simulink model "Inverter"  (Simulink 8.3)
settings: Solver=ode45  StartTime=0.0  StopTime=tfin  RelTol=1e-3
values from neighbouring files (symbols this model uses):
  Bridge_Inductances = 4e-3    (= 0.004)    [Inverter_ini.m]
  Buffer_Capacitance = 10e-3    (= 0.01)    [Inverter_ini.m]
  sample = 10e-5    (= 0.0001)    [Inverter_ini.m]    (also in Sketch_controller_model_ini.m; Symmetry_REAL_TIME_ini.m; Symmetry_ini.m; Symmetry_ini_COPY.m)
undefined symbols (not defined in the file or in its folder): Ion, Lithium
libraries: powerlib x69, simulink x5, dspsigops x4, dsparch4 x2, electricdrivelib x1
settings Model: Creator=gorbep  LastModifiedBy=Templomos
settings DataIOCC: SignalLoggingSaveFormat=Dataset
settings DebuggingCC: UnderspecifiedInitializationDetection=Simplified  StateNameClashWarn=none
settings GRTTargetCC: CombineOutputUpdateFcns=on  GRTInterface=off

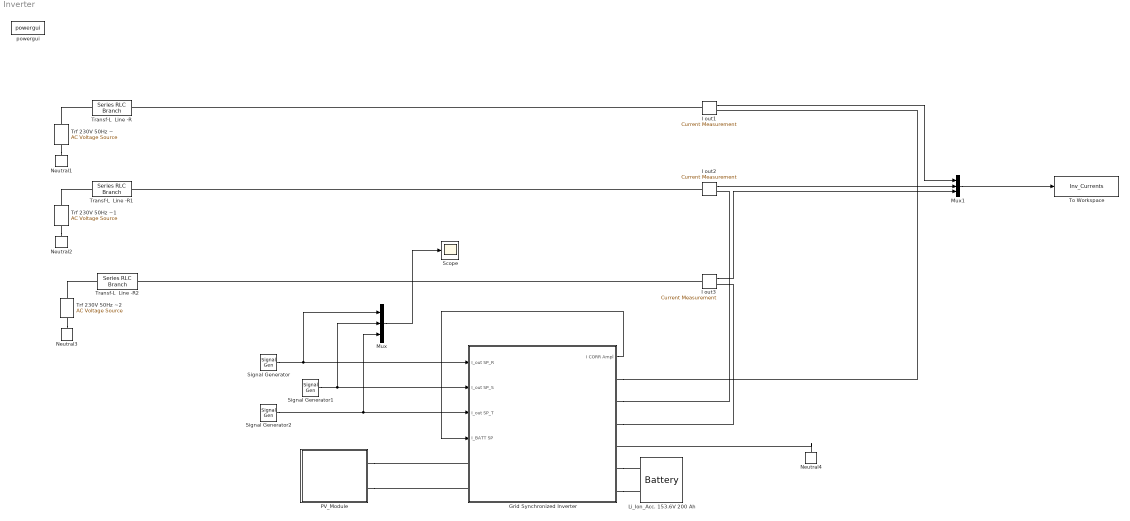
== system Inverter ==
  Grid Synchronized Inverter : Subsystem
  I out1 : powerlib/Measurements/Current Measurement  PhasorSimulation=off  OutputType=Complex  PSBequivalent=0
  I out2 : powerlib/Measurements/Current Measurement  PhasorSimulation=off  OutputType=Complex  PSBequivalent=0
  I out3 : powerlib/Measurements/Current Measurement  PhasorSimulation=off  OutputType=Complex  PSBequivalent=0
  Li_Ion_Acc. 153.6V 200 Ah : electricdrivelib/Extra Sources/Battery  BatType=Lithium-Ion  ShowDetailedParameters=off  NomV=153.6  NomQ=200  SOC=50  PresetModel=off  MaxQ=210  FullV=274.6189824  Dis_rate=173.913  R=0.00768  Normal_OP=361.7392  expZone=[254.8950528 19.652174]  Dis_Char=off  current=[1.5 3]  Units=Ampere-hour  Batt_Tr=30
  Mux : Mux  Inputs=3
  Mux1 : Mux  Inputs=3
  Neutral{1..4} (4 alike) : powerlib/Elements/Neutral  LConnTagsString=a  NodeNumber=10
  PV_Module : Subsystem
  Scope : Scope
      settings: SaveName=ScopeData5
  Signal Generator : SignalGenerator  WaveForm=sawtooth  Frequency=200
  Signal Generator1 : SignalGenerator  WaveForm=square  Frequency=200
  Signal Generator2 : SignalGenerator  Frequency=200
  To Workspace : ToWorkspace  VariableName=Inv_Currents  SaveFormat=Structure With Time  SampleTime=sample
  Transf-L  Line -R : powerlib/Elements/Series RLC Branch  LConnTagsString=__new0  RConnTagsString=__new0  BranchType=RL  Resistance=0.01  Inductance=0  SetiL0=off  InitialCurrent=0  Capacitance=1.0  Setx0=off  InitialVoltage=0  Measurements=None
  Transf-L  Line -R1 : powerlib/Elements/Series RLC Branch  LConnTagsString=__new0  RConnTagsString=__new0  BranchType=RL  Resistance=0.01  Inductance=0  SetiL0=off  InitialCurrent=0  Capacitance=1.0  Setx0=off  InitialVoltage=0  Measurements=None
  Transf-L  Line -R2 : powerlib/Elements/Series RLC Branch  LConnTagsString=__new0  RConnTagsString=__new0  BranchType=RL  Resistance=0.01  Inductance=0  SetiL0=off  InitialCurrent=0  Capacitance=1.0  Setx0=off  InitialVoltage=0  Measurements=None
  Trf 230V 50Hz ~ : powerlib/Electrical Sources/AC Voltage Source  Amplitude=325.2691  Phase=0  Frequency=50  SampleTime=0  Measurements=None
  Trf 230V 50Hz ~1 : powerlib/Electrical Sources/AC Voltage Source  Amplitude=325.2691  Phase=-120  Frequency=50  SampleTime=0  Measurements=None
  Trf 230V 50Hz ~2 : powerlib/Electrical Sources/AC Voltage Source  Amplitude=325.2691  Phase=-240  Frequency=50  SampleTime=0  Measurements=None
  powergui : powerlib/powergui  SimulationMode=Continuous  SolverType=Tustin  SampleTime=50e-6  frequency=60  SPID=off  DisableSnubberDevices=off  DisableRonSwitches=off  DisableVfSwitches=off  SwTol=0  Interpol=off  DisplayEquations=off  Ts=0  methode=off  frequencyindice=50  Pbase=100e6  ErrMax=1e-4  Iterations=50  UnitsV=kV  UnitsW=MW  FunctionMessages=off  echomessages=off  HookPort=off  EnableUseOfTLC=off  x0status=blocks  RestoreLinks=warning  ResistiveCurrentMeasurement=off  Frange=[0:2:500]  Ylog=off  Xlog=on  ShowGrid=off  save=off  variable=ZData  structure=0  ZoomFFT=on  StartTime=0.0  cycles=1  DisplayStyle=1  fundamental=60  FreqAxis=off  MaxFrequency=1000  frequencyindicesteady=1  RmsSteady=1  display=off
  wires:
  Grid Synchronized Inverter/1(I CORR Ampl) -> Grid Synchronized Inverter/4(I_BATT SP)
  Signal Generator/1 -> Mux/1, Grid Synchronized Inverter/1(I_out SP_R)
  Signal Generator1/1 -> Mux/2, Grid Synchronized Inverter/2(I_out SP_S)
  Signal Generator2/1 -> Mux/3, Grid Synchronized Inverter/3(I_out SP_T)
  I out1/1 -> Mux1/1
  I out2/1 -> Mux1/2
  I out3/1 -> Mux1/3
  Mux1/1 -> To Workspace/1
  Mux/1 -> Scope/1
  connections:
  Grid Synchronized Inverter/RConn5 -- Li_Ion_Acc. 153.6V 200 Ah/LConn1
  Grid Synchronized Inverter/RConn6 -- Li_Ion_Acc. 153.6V 200 Ah/LConn2
  Transf-L  Line -R/LConn1 -- Trf 230V 50Hz ~/RConn1
  Trf 230V 50Hz ~/LConn1 -- Neutral1/LConn1
  Transf-L  Line -R1/LConn1 -- Trf 230V 50Hz ~1/RConn1
  Trf 230V 50Hz ~1/LConn1 -- Neutral2/LConn1
  Trf 230V 50Hz ~2/LConn1 -- Neutral3/LConn1
  Transf-L  Line -R2/LConn1 -- Trf 230V 50Hz ~2/RConn1
  I out1/LConn1 -- Transf-L  Line -R/RConn1
  I out2/LConn1 -- Transf-L  Line -R1/RConn1
  I out3/LConn1 -- Transf-L  Line -R2/RConn1
  Neutral4/LConn1 -- Grid Synchronized Inverter/RConn4
  Grid Synchronized Inverter/RConn1 -- I out1/RConn1
  Grid Synchronized Inverter/RConn2 -- I out2/RConn1
  Grid Synchronized Inverter/RConn3 -- I out3/RConn1
  PV_Module/RConn1 -- Grid Synchronized Inverter/LConn1
  PV_Module/RConn2 -- Grid Synchronized Inverter/LConn2

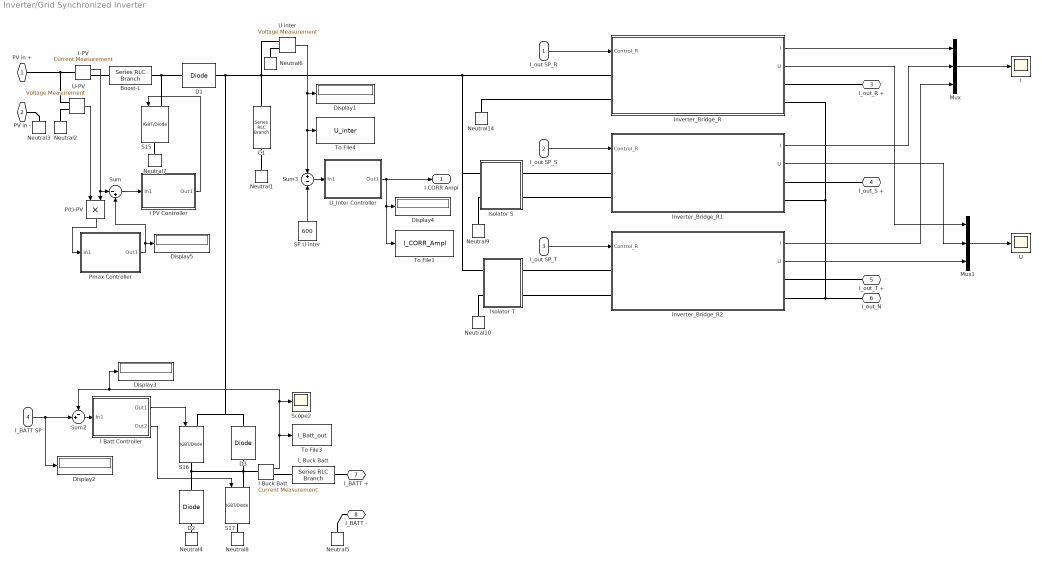
== system Inverter/Grid Synchronized Inverter ==
  I_out SP_R : Inport
  I_out SP_S : Inport  Port=2
  I_out SP_T : Inport  Port=3
  I_BATT SP : Inport  Port=4
  " Boost-L" : powerlib/Elements/Series RLC Branch  LConnTagsString=__new0  RConnTagsString=__new0  BranchType=L  Resistance=8  Inductance=100e-3  SetiL0=off  InitialCurrent=30  Capacitance=1.0  Setx0=off  InitialVoltage=0  Measurements=None
  C1 : powerlib/Elements/Series RLC Branch  LConnTagsString=__new0  RConnTagsString=__new0  BranchType=C  Resistance=35.35  Inductance=0.1125  SetiL0=off  InitialCurrent=0  Capacitance=Buffer_Capacitance  Setx0=on  InitialVoltage=Buffer_Initial_Voltage  Measurements=None
  D1 : powerlib/Power Electronics/Diode  Ron=0.001  Lon=0  Vf=0.8  IC=0  UseSnubber=off  Rs=50000  Cs=250e-9  Measurements=off
  D2 : powerlib/Power Electronics/Diode  Ron=0.001  Lon=0  Vf=0.8  IC=0  UseSnubber=off  Rs=50000  Cs=250e-9  Measurements=off
  D3 : powerlib/Power Electronics/Diode  Ron=0.001  Lon=0  Vf=0.8  IC=0  UseSnubber=off  Rs=50000  Cs=250e-9  Measurements=off
  Display{1..5} (5 alike) : Display
  I : Scope
      settings: YMin=-550  YMax=400
  I Batt Controller : Subsystem
  I Buck Batt : powerlib/Measurements/Current Measurement  PhasorSimulation=off  OutputType=Complex  PSBequivalent=0
  I PV Controller : Subsystem
  I-PV : powerlib/Measurements/Current Measurement  PhasorSimulation=off  OutputType=Complex  PSBequivalent=0
  Inverter_Bridge_R : Subsystem
  Inverter_Bridge_R1 : Subsystem
  Inverter_Bridge_R2 : Subsystem
  Isolator S : Subsystem
  Isolator T : Subsystem
  L Buck Batt : powerlib/Elements/Series RLC Branch  LConnTagsString=__new0  RConnTagsString=__new0  BranchType=L  Resistance=100  Inductance=1e-1  SetiL0=on  InitialCurrent=0  Capacitance=1.0  Setx0=off  InitialVoltage=0  Measurements=None
  Mux : Mux  Inputs=3
  Mux1 : Mux  Inputs=3
  Neutral{1..10,14} (11 alike) : powerlib/Elements/Neutral  LConnTagsString=a  NodeNumber=1
  P(t)-PV : Product  RndMeth=Zero
  Pmax Controller : Subsystem
  S15 : powerlib/Power Electronics/IGBT//Diode  Ron=1e-3  Rs=1e5  Cs=inf  Measurements=off
  S16 : powerlib/Power Electronics/IGBT//Diode  Ron=1e-3  Rs=1e5  Cs=inf  Measurements=off
  S17 : powerlib/Power Electronics/IGBT//Diode  Ron=1e-3  Rs=1e5  Cs=inf  Measurements=off
  SP U inter : Constant  Value=600
  Scope2 : Scope
      settings: TimeRange=0.1  YMin=-40  YMax=40  SaveName=ScopeData2
  Sum : Sum  Inputs=|-+
  Sum2 : Sum  Inputs=-+|
  Sum3 : Sum  Inputs=+-
  To File1 : ToFile  Filename=I_CORR_Ampl  MatrixName=y  SampleTime=5e-3
  To File3 : ToFile  Filename=I_Batt_out  MatrixName=y  SampleTime=5e-3
  To File4 : ToFile  Filename=U_inter  MatrixName=y  SampleTime=5e-3
  U : Scope
      settings: YMin=-1.1  YMax=1.1
  U inter : powerlib/Measurements/Voltage Measurement  PhasorSimulation=off  OutputType=Complex  PSBequivalent=0
  U-PV : powerlib/Measurements/Voltage Measurement  PhasorSimulation=off  OutputType=Complex  PSBequivalent=0
  U_Inter Controller : Subsystem
  " PV in +" : PMIOPort  Port=1  Side=Left
  " PV in -" : PMIOPort  Port=2  Side=Left
  " I_out_R +" : PMIOPort  Port=3  Side=Right
  " I_out_S +" : PMIOPort  Port=4  Side=Right
  " I_out_T +" : PMIOPort  Port=5  Side=Right
  " I_out_N" : PMIOPort  Port=6  Side=Right
  " I_BATT +" : PMIOPort  Port=7  Side=Right
  " I_BATT -" : PMIOPort  Port=8  Side=Right
  I CORR Ampl : Outport
  wires:
  U inter/1 -> Sum3/1, To File4/1, Display1/1
  Sum/1 -> I PV Controller/1(In1)
  I-PV/1 -> Sum/1, P(t)-PV/2
  SP U inter/1 -> Sum3/2
  U-PV/1 -> P(t)-PV/1
  Pmax Controller/1(Out1) -> Display5/1, Sum/2
  I PV Controller/1(Out1) -> S15/1
  P(t)-PV/1 -> Pmax Controller/1(In1)
  U_Inter Controller/1(Out1) -> I CORR Ampl/1, To File1/1, Display4/1
  Sum3/1 -> U_Inter Controller/1(In1)
  Sum2/1 -> I Batt Controller/1(In1)
  I Buck Batt/1 -> To File3/1, Scope2/1, Sum2/1, Display3/1
  I Batt Controller/1(Out1) -> S16/1
  I_BATT SP/1 -> Sum2/2, Display2/1
  I Batt Controller/2(Out2) -> S17/1
  I_out SP_R/1 -> Inverter_Bridge_R/1(Control_R)
  I_out SP_S/1 -> Inverter_Bridge_R1/1(Control_R)
  I_out SP_T/1 -> Inverter_Bridge_R2/1(Control_R)
  Inverter_Bridge_R/1(I) -> Mux/1
  Inverter_Bridge_R1/1(I) -> Mux/2
  Inverter_Bridge_R2/1(I) -> Mux/3
  Mux1/1 -> U/1
  Inverter_Bridge_R2/2(U) -> Mux1/3
  Inverter_Bridge_R1/2(U) -> Mux1/2
  Inverter_Bridge_R/2(U) -> Mux1/1
  Mux/1 -> I/1
  connections:
  " Boost-L"/RConn1 -- D1/LConn1 -- S15/LConn1
  " PV in +"/RConn1 -- I-PV/LConn1 -- U-PV/LConn1
  Neutral6/LConn1 -- U inter/LConn2
  Neutral7/LConn1 -- S15/RConn1
  I-PV/RConn1 -- " Boost-L"/LConn1
  Neutral1/LConn1 -- C1/RConn1
  U-PV/LConn2 -- Neutral2/LConn1
  " PV in -"/RConn1 -- Neutral3/LConn1
  I Buck Batt/LConn1 -- S17/LConn1 -- D3/LConn1 -- S16/RConn1 -- D2/RConn1
  Neutral4/LConn1 -- D2/LConn1
  L Buck Batt/RConn1 -- " I_BATT +"/RConn1
  Neutral5/LConn1 -- " I_BATT -"/RConn1
  S17/RConn1 -- Neutral8/LConn1
  I Buck Batt/RConn1 -- L Buck Batt/LConn1
  C1/LConn1 -- Isolator T/RConn1 -- Isolator S/RConn1 -- Inverter_Bridge_R/LConn1 -- D3/RConn1 -- S16/LConn1 -- D1/RConn1 -- U inter/LConn1
  Neutral10/LConn1 -- Isolator T/RConn2
  Neutral9/LConn1 -- Isolator S/RConn2
  " I_out_R +"/RConn1 -- Inverter_Bridge_R/RConn1
  Inverter_Bridge_R/LConn2 -- Neutral14/LConn1
  Inverter_Bridge_R1/LConn1 -- Isolator S/LConn1
  Inverter_Bridge_R1/LConn2 -- Isolator S/LConn2
  Inverter_Bridge_R1/RConn1 -- " I_out_S +"/RConn1
  " I_out_N"/RConn1 -- Inverter_Bridge_R2/RConn2 -- Inverter_Bridge_R1/RConn2 -- Inverter_Bridge_R/RConn2
  Inverter_Bridge_R2/LConn1 -- Isolator T/LConn1
  Inverter_Bridge_R2/LConn2 -- Isolator T/LConn2
  Inverter_Bridge_R2/RConn1 -- " I_out_T +"/RConn1

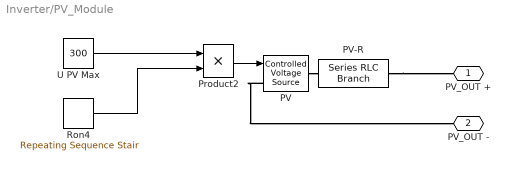
== system Inverter/PV_Module ==
  PV : powerlib/Electrical Sources/Controlled Voltage Source  Initialize=off  Source_Type=AC  Amplitude=0  Phase=0  Frequency=0  Measurements=None
  PV-R : powerlib/Elements/Series RLC Branch  LConnTagsString=__new0  RConnTagsString=__new0  BranchType=R  Resistance=5  Inductance=0.1  SetiL0=off  InitialCurrent=0  Capacitance=1.0  Setx0=off  InitialVoltage=0  Measurements=None
  Product2 : Product  RndMeth=Zero
  Ron4 : simulink/Sources/Repeating Sequence Stair  OutValues=[1 1 0 0].'  tsamp=0.5  OutMin=[]  OutMax=[]  OutDataTypeStr=float('double')  OutputDataTypeScalingMode=Specify via dialog  OutDataType=float('double')  ConRadixGroup=Best Precision: Vector-wise  OutScaling=2^-12
  U PV Max : Constant  Value=300
  PV_OUT + : PMIOPort  Port=1  Side=Right
  PV_OUT - : PMIOPort  Port=2  Side=Right
  wires:
  Product2/1 -> PV/1
  U PV Max/1 -> Product2/1
  Ron4/1 -> Product2/2
  connections:
  PV/LConn1 -- PV_OUT -/RConn1
  PV/RConn1 -- PV-R/LConn1
  PV-R/RConn1 -- PV_OUT +/RConn1

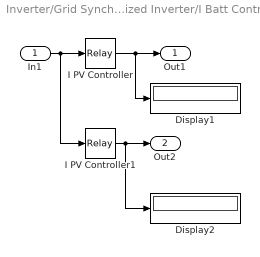
== system Inverter/Grid Synchronized Inverter/I Batt Controller ==
  In1 : Inport
  Display1 : Display
  Display2 : Display
  I PV Controller : Relay  OnSwitchValue=0.01  OffSwitchValue=-0.01  ZeroCross=off  SampleTime=1e-4
  I PV Controller1 : Relay  OnSwitchValue=0.01  OffSwitchValue=-0.01  OnOutputValue=0  OffOutputValue=1  ZeroCross=off  SampleTime=1e-4
  Out1 : Outport
  Out2 : Outport  Port=2
  wires:
  In1/1 -> I PV Controller/1, I PV Controller1/1
  I PV Controller/1 -> Out1/1, Display1/1
  I PV Controller1/1 -> Out2/1, Display2/1

== system Inverter/Grid Synchronized Inverter/I PV Controller ==
  In1 : Inport
  I PV Controller : Relay  OnSwitchValue=0.01  OffSwitchValue=-0.01  ZeroCross=off  SampleTime=1e-4
  Out1 : Outport
  wires:
  In1/1 -> I PV Controller/1
  I PV Controller/1 -> Out1/1

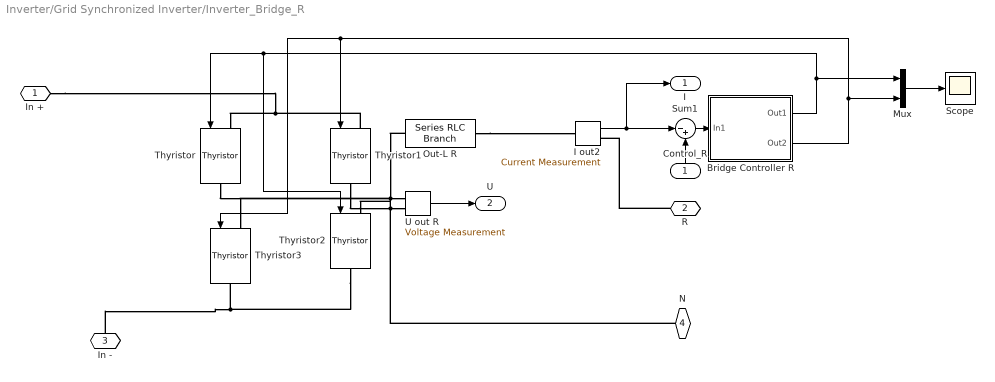
== system Inverter/Grid Synchronized Inverter/Inverter_Bridge_R ==
  Control_R : Inport
  " Out-L R" : powerlib/Elements/Series RLC Branch  LConnTagsString=__new0  RConnTagsString=__new0  BranchType=L  Resistance=100  Inductance=Bridge_Inductances  SetiL0=off  InitialCurrent=0  Capacitance=1.0  Setx0=off  InitialVoltage=0  Measurements=None
  Bridge Controller R : Subsystem
  I out2 : powerlib/Measurements/Current Measurement  PhasorSimulation=off  OutputType=Complex  PSBequivalent=0
  Mux : Mux  Inputs=2
  Scope : Scope
      settings: SaveName=ScopeData4
  Sum1 : Sum  Inputs=|-+
  Thyristor{,1..3} (4 alike) : powerlib/Power Electronics/Thyristor  Ron=1e-3  Lon=0  Vf=0.8  IC=0  Rs=500  Cs=inf  Measurements=off
  U out R : powerlib/Measurements/Voltage Measurement  PhasorSimulation=off  OutputType=Complex  PSBequivalent=0
  In + : PMIOPort  Port=1  Side=Left
  R : PMIOPort  Port=2  Side=Right
  In - : PMIOPort  Port=3  Side=Left
  N : PMIOPort  Port=4  Side=Right
  I : Outport
  U : Outport  Port=2
  wires:
  I out2/1 -> I/1, Sum1/1
  Bridge Controller R/2(Out2) -> Mux/2, Thyristor1/1, Thyristor3/1
  Bridge Controller R/1(Out1) -> Mux/1, Thyristor2/1, Thyristor/1
  Sum1/1 -> Bridge Controller R/1(In1)
  Control_R/1 -> Sum1/2
  U out R/1 -> U/1
  Mux/1 -> Scope/1
  connections:
  U out R/LConn1 -- Thyristor/RConn1 -- Thyristor3/LConn1 -- " Out-L R"/LConn1
  " Out-L R"/RConn1 -- I out2/LConn1
  R/RConn1 -- I out2/RConn1
  In +/RConn1 -- Thyristor1/LConn1 -- Thyristor/LConn1
  N/RConn1 -- Thyristor1/RConn1 -- Thyristor2/LConn1 -- U out R/LConn2
  In -/RConn1 -- Thyristor2/RConn1 -- Thyristor3/RConn1

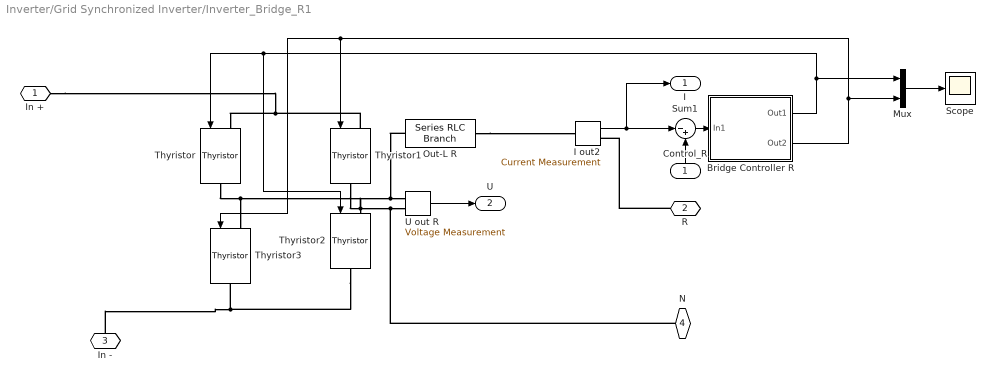
== system Inverter/Grid Synchronized Inverter/Inverter_Bridge_R1 ==
  Control_R : Inport
  " Out-L R" : powerlib/Elements/Series RLC Branch  LConnTagsString=__new0  RConnTagsString=__new0  BranchType=L  Resistance=100  Inductance=Bridge_Inductances  SetiL0=off  InitialCurrent=0  Capacitance=1.0  Setx0=off  InitialVoltage=0  Measurements=None
  Bridge Controller R : Subsystem
  I out2 : powerlib/Measurements/Current Measurement  PhasorSimulation=off  OutputType=Complex  PSBequivalent=0
  Mux : Mux  Inputs=2
  Scope : Scope
      settings: SaveName=ScopeData4
  Sum1 : Sum  Inputs=|-+
  Thyristor{,1..3} (4 alike) : powerlib/Power Electronics/Thyristor  Ron=1e-3  Lon=0  Vf=0.8  IC=0  Rs=500  Cs=inf  Measurements=off
  U out R : powerlib/Measurements/Voltage Measurement  PhasorSimulation=off  OutputType=Complex  PSBequivalent=0
  In + : PMIOPort  Port=1  Side=Left
  R : PMIOPort  Port=2  Side=Right
  In - : PMIOPort  Port=3  Side=Left
  N : PMIOPort  Port=4  Side=Right
  I : Outport
  U : Outport  Port=2
  wires:
  Mux/1 -> Scope/1
  U out R/1 -> U/1
  Control_R/1 -> Sum1/2
  Sum1/1 -> Bridge Controller R/1(In1)
  Bridge Controller R/1(Out1) -> Thyristor/1, Thyristor2/1, Mux/1
  Bridge Controller R/2(Out2) -> Thyristor3/1, Thyristor1/1, Mux/2
  I out2/1 -> Sum1/1, I/1
  connections:
  Thyristor3/RConn1 -- In -/RConn1 -- Thyristor2/RConn1
  Thyristor2/LConn1 -- U out R/LConn2 -- N/RConn1 -- Thyristor1/RConn1
  Thyristor1/LConn1 -- In +/RConn1 -- Thyristor/LConn1
  R/RConn1 -- I out2/RConn1
  " Out-L R"/RConn1 -- I out2/LConn1
  Thyristor3/LConn1 -- Thyristor/RConn1 -- " Out-L R"/LConn1 -- U out R/LConn1

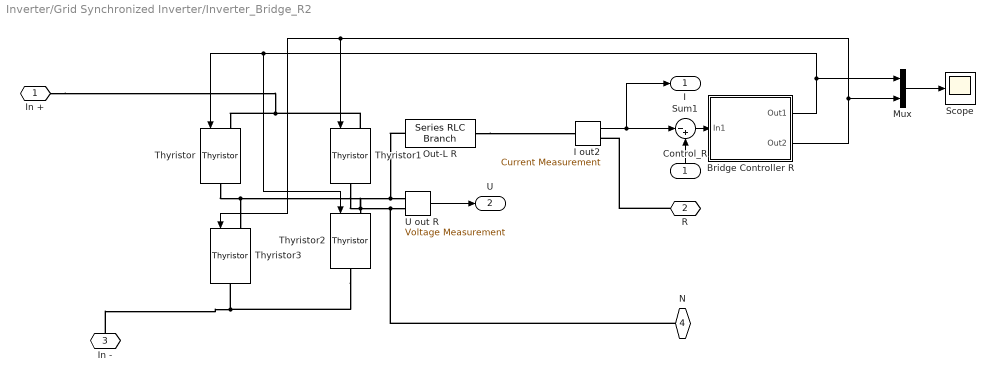
== system Inverter/Grid Synchronized Inverter/Inverter_Bridge_R2 ==
  Control_R : Inport
  " Out-L R" : powerlib/Elements/Series RLC Branch  LConnTagsString=__new0  RConnTagsString=__new0  BranchType=L  Resistance=100  Inductance=Bridge_Inductances  SetiL0=off  InitialCurrent=0  Capacitance=1.0  Setx0=off  InitialVoltage=0  Measurements=None
  Bridge Controller R : Subsystem
  I out2 : powerlib/Measurements/Current Measurement  PhasorSimulation=off  OutputType=Complex  PSBequivalent=0
  Mux : Mux  Inputs=2
  Scope : Scope
      settings: SaveName=ScopeData4
  Sum1 : Sum  Inputs=|-+
  Thyristor{,1..3} (4 alike) : powerlib/Power Electronics/Thyristor  Ron=1e-3  Lon=0  Vf=0.8  IC=0  Rs=500  Cs=inf  Measurements=off
  U out R : powerlib/Measurements/Voltage Measurement  PhasorSimulation=off  OutputType=Complex  PSBequivalent=0
  In + : PMIOPort  Port=1  Side=Left
  R : PMIOPort  Port=2  Side=Right
  In - : PMIOPort  Port=3  Side=Left
  N : PMIOPort  Port=4  Side=Right
  I : Outport
  U : Outport  Port=2
  wires:
  Mux/1 -> Scope/1
  U out R/1 -> U/1
  Control_R/1 -> Sum1/2
  Sum1/1 -> Bridge Controller R/1(In1)
  Bridge Controller R/1(Out1) -> Thyristor/1, Thyristor2/1, Mux/1
  Bridge Controller R/2(Out2) -> Thyristor3/1, Thyristor1/1, Mux/2
  I out2/1 -> Sum1/1, I/1
  connections:
  Thyristor3/RConn1 -- In -/RConn1 -- Thyristor2/RConn1
  Thyristor2/LConn1 -- U out R/LConn2 -- N/RConn1 -- Thyristor1/RConn1
  Thyristor1/LConn1 -- In +/RConn1 -- Thyristor/LConn1
  R/RConn1 -- I out2/RConn1
  " Out-L R"/RConn1 -- I out2/LConn1
  Thyristor3/LConn1 -- Thyristor/RConn1 -- " Out-L R"/LConn1 -- U out R/LConn1

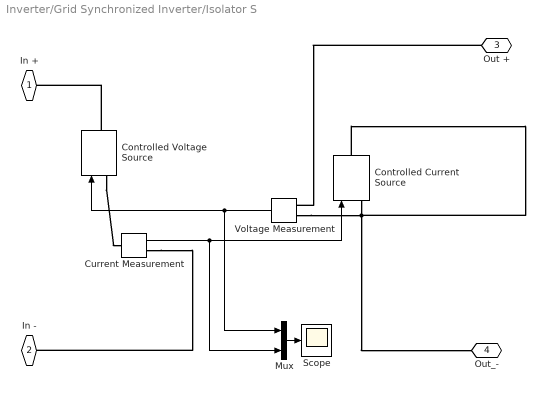
== system Inverter/Grid Synchronized Inverter/Isolator S ==
  Controlled Current Source : powerlib/Electrical Sources/Controlled Current Source  Initialize=on  Source_Type=AC  Amplitude=0  Phase=0  Frequency=0  Measurements=None
  Controlled Voltage Source : powerlib/Electrical Sources/Controlled Voltage Source  Initialize=on  Source_Type=AC  Amplitude=0  Phase=0  Frequency=0  Measurements=None
  Current Measurement : powerlib/Measurements/Current Measurement  PhasorSimulation=off  OutputType=Complex  PSBequivalent=0
  Mux : Mux  Inputs=2
  Scope : Scope
      settings: TimeRange=0.002  YMin=-600000  YMax=100000  SaveName=ScopeData3
  Voltage Measurement : powerlib/Measurements/Voltage Measurement  PhasorSimulation=off  OutputType=Complex  PSBequivalent=0
  In + : PMIOPort  Port=1  Side=Left
  " In -" : PMIOPort  Port=2  Side=Left
  " Out +" : PMIOPort  Port=3  Side=Right
  " Out_-" : PMIOPort  Port=4  Side=Right
  wires:
  Voltage Measurement/1 -> Mux/1, Controlled Voltage Source/1
  Current Measurement/1 -> Mux/2, Controlled Current Source/1
  Mux/1 -> Scope/1
  connections:
  Controlled Voltage Source/RConn1 -- In +/RConn1
  Controlled Voltage Source/LConn1 -- Current Measurement/LConn1
  Current Measurement/RConn1 -- " In -"/RConn1
  Controlled Current Source/LConn1 -- Controlled Current Source/RConn1 -- Voltage Measurement/LConn2 -- " Out_-"/RConn1
  " Out +"/RConn1 -- Voltage Measurement/LConn1

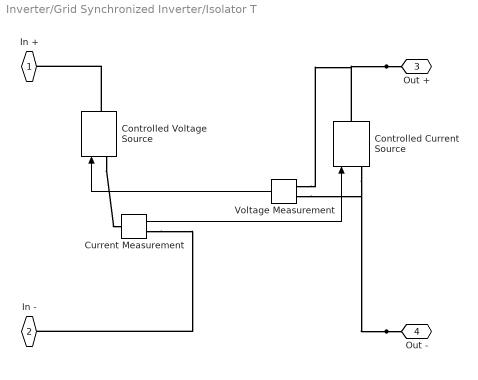
== system Inverter/Grid Synchronized Inverter/Isolator T ==
  Controlled Current Source : powerlib/Electrical Sources/Controlled Current Source  Initialize=on  Source_Type=AC  Amplitude=0  Phase=0  Frequency=0  Measurements=None
  Controlled Voltage Source : powerlib/Electrical Sources/Controlled Voltage Source  Initialize=on  Source_Type=AC  Amplitude=0  Phase=0  Frequency=0  Measurements=None
  Current Measurement : powerlib/Measurements/Current Measurement  PhasorSimulation=off  OutputType=Complex  PSBequivalent=0
  Voltage Measurement : powerlib/Measurements/Voltage Measurement  PhasorSimulation=off  OutputType=Complex  PSBequivalent=0
  In + : PMIOPort  Port=1  Side=Left
  " In -" : PMIOPort  Port=2  Side=Left
  " Out +" : PMIOPort  Port=3  Side=Right
  " Out -" : PMIOPort  Port=4  Side=Right
  wires:
  Voltage Measurement/1 -> Controlled Voltage Source/1
  Current Measurement/1 -> Controlled Current Source/1
  connections:
  Controlled Voltage Source/RConn1 -- In +/RConn1
  Controlled Voltage Source/LConn1 -- Current Measurement/LConn1
  Current Measurement/RConn1 -- " In -"/RConn1
  " Out +"/RConn1 -- Controlled Current Source/RConn1 -- Voltage Measurement/LConn1
  " Out -"/RConn1 -- Controlled Current Source/LConn1 -- Voltage Measurement/LConn2

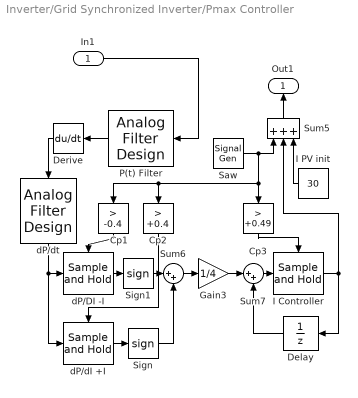
== system Inverter/Grid Synchronized Inverter/Pmax Controller ==
  In1 : Inport
  Cp1 : simulink/Logic and Bit Operations/Compare To Constant  relop=>  const=-0.4  OutDataTypeStr=uint8  ZeroCross=off
  Cp2 : simulink/Logic and Bit Operations/Compare To Constant  relop=>  const=+0.4  OutDataTypeStr=uint8  ZeroCross=off
  Cp3 : simulink/Logic and Bit Operations/Compare To Constant  relop=>  const=+0.49  OutDataTypeStr=uint8  ZeroCross=off
  Delay : UnitDelay  SampleTime=0.01
  Derive : Derivative
  Gain3 : Gain  Gain=1/4
  I Controller : dspsigops/Sample and Hold  trig=Rising edge  initCond=0  latchinput=off
  "I PV init " : Constant  Value=30
  P(t) Filter : dsparch4/Analog Filter Design  method=Butterworth  filttype=Lowpass  N=1  Wlo=628  Whi=80  Rp=2  Rs=40
  Saw : SignalGenerator  WaveForm=sawtooth  Amplitude=-0.5  Frequency=10
  Sign : Signum
  Sign1 : Signum
  Sum5 : Sum  Inputs=+++
  Sum6 : Sum  Inputs=|++
  Sum7 : Sum  Inputs=|++
  dP/DI -I : dspsigops/Sample and Hold  trig=Rising edge  initCond=0  latchinput=off
  dP/dI +I : dspsigops/Sample and Hold  trig=Rising edge  initCond=0  latchinput=off
  "dP/dt " : dsparch4/Analog Filter Design  method=Butterworth  filttype=Lowpass  N=8  Wlo=6280  Whi=80  Rp=2  Rs=40
  Out1 : Outport
  wires:
  P(t) Filter/1 -> Derive/1
  I Controller/1 -> Sum5/2, Delay/1
  "I PV init "/1 -> Sum5/3
  Sign1/1 -> Sum6/1
  dP/DI -I/1 -> Sign1/1
  Sign/1 -> Sum6/2
  dP/dI +I/1 -> Sign/1
  Delay/1 -> Sum7/2
  Saw/1 -> Sum5/1, Cp3/1, Cp2/1, Cp1/1
  Cp3/1 -> I Controller/Trigger
  Sum7/1 -> I Controller/1
  Gain3/1 -> Sum7/1
  Sum6/1 -> Gain3/1
  Cp2/1 -> dP/dI +I/Trigger
  Cp1/1 -> dP/DI -I/Trigger
  "dP/dt "/1 -> dP/DI -I/1, dP/dI +I/1
  Derive/1 -> "dP/dt "/1
  Sum5/1 -> Out1/1
  In1/1 -> P(t) Filter/1

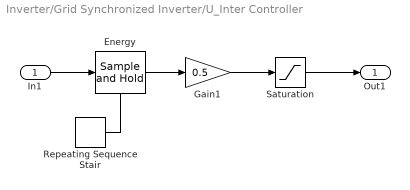
== system Inverter/Grid Synchronized Inverter/U_Inter Controller ==
  In1 : Inport
  Energy : dspsigops/Sample and Hold  trig=Rising edge  initCond=18  latchinput=off
  Gain1 : Gain  Gain=0.5
  Repeating Sequence Stair : simulink/Sources/Repeating Sequence Stair  OutValues=[ 1 0 ]  tsamp=0.01  OutMin=[]  OutMax=[]  OutDataTypeStr=float('double')  OutputDataTypeScalingMode=Specify via dialog  OutDataType=float('double')  ConRadixGroup=Best Precision: Vector-wise  OutScaling=2^-12
  Saturation : Saturate  UpperLimit=50  LowerLimit=-50
  Out1 : Outport
  wires:
  Gain1/1 -> Saturation/1
  Saturation/1 -> Out1/1
  In1/1 -> Energy/1
  Energy/1 -> Gain1/1
  Repeating Sequence Stair/1 -> Energy/Trigger

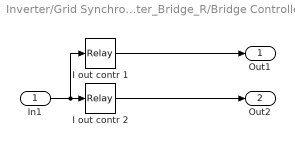
== system Inverter/Grid Synchronized Inverter/Inverter_Bridge_R/Bridge Controller R ==
  In1 : Inport
  I out contr 1 : Relay  OnSwitchValue=0.01  OffSwitchValue=-0.01  OnOutputValue=10  ZeroCross=off  SampleTime=1e-6
  I out contr 2 : Relay  OnSwitchValue=0.01  OffSwitchValue=-0.01  OnOutputValue=0  OffOutputValue=10  ZeroCross=off  SampleTime=1e-6
  Out1 : Outport
  Out2 : Outport  Port=2
  wires:
  In1/1 -> I out contr 1/1, I out contr 2/1
  I out contr 1/1 -> Out1/1
  I out contr 2/1 -> Out2/1

== system Inverter/Grid Synchronized Inverter/Inverter_Bridge_R1/Bridge Controller R ==
  In1 : Inport
  I out contr 1 : Relay  OnSwitchValue=0.01  OffSwitchValue=-0.01  OnOutputValue=10  ZeroCross=off  SampleTime=1e-6
  I out contr 2 : Relay  OnSwitchValue=0.01  OffSwitchValue=-0.01  OnOutputValue=0  OffOutputValue=10  ZeroCross=off  SampleTime=1e-6
  Out1 : Outport
  Out2 : Outport  Port=2
  wires:
  I out contr 2/1 -> Out2/1
  I out contr 1/1 -> Out1/1
  In1/1 -> I out contr 2/1, I out contr 1/1

== system Inverter/Grid Synchronized Inverter/Inverter_Bridge_R2/Bridge Controller R ==
  In1 : Inport
  I out contr 1 : Relay  OnSwitchValue=0.01  OffSwitchValue=-0.01  OnOutputValue=10  ZeroCross=off  SampleTime=1e-6
  I out contr 2 : Relay  OnSwitchValue=0.01  OffSwitchValue=-0.01  OnOutputValue=0  OffOutputValue=10  ZeroCross=off  SampleTime=1e-6
  Out1 : Outport
  Out2 : Outport  Port=2
  wires:
  I out contr 2/1 -> Out2/1
  I out contr 1/1 -> Out1/1
  In1/1 -> I out contr 2/1, I out contr 1/1
